simulink model "SimPendulo"  (R2023b)
settings: Solver=VariableStepAuto  StartTime=0.0  StopTime=10.0  RelTol=1e-3
settings Model: Creator=mluser  LastModifiedBy=mluser

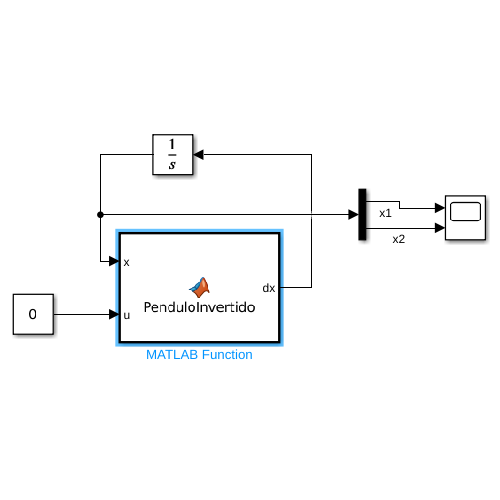
[thumbnail: Simulink's stored preview of the top-level diagram]
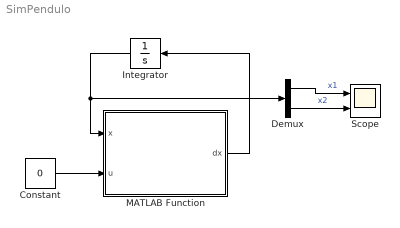
== system SimPendulo ==
  Constant : Constant  Value=0
  Demux : Demux  Outputs=2
  Integrator : Integrator  InitialCondition=[0.1; 0]
  MATLAB Function : MATLAB Function  TreatAsAtomicUnit=on
  Scope : Scope  NumInputPorts=2
  wires:
  MATLAB Function/1(dx) -> Integrator/1
  Integrator/1 -> Demux/1, MATLAB Function/1(x)
  Constant/1 -> MATLAB Function/2(u)
  Demux/1 -> Scope/1  "x1"
  Demux/2 -> Scope/2  "x2"

== matlab function SimPendulo/MATLAB Function ==
  data: x input; u input; dx output
function dx = PenduloInvertido(x,u)
%Definicin de Parmetros
m=1; g=9.81; L=1; b=2; J=m*L^2;

%definicin de Variables
x1 = x(1);
x2 = x(2);

dx = [x2;...
     m*g*L/J*sin(x1)-b/J*x2+1/J*u];
